simulink model "orthosis_robust"  (R2017b)
settings: Solver=ode45  StartTime=0.0  StopTime=40  RelTol=1e-3
settings Model: SimulationMode=accelerator  Creator=ArsalanBangash  LastModifiedBy=ArsalanBangash

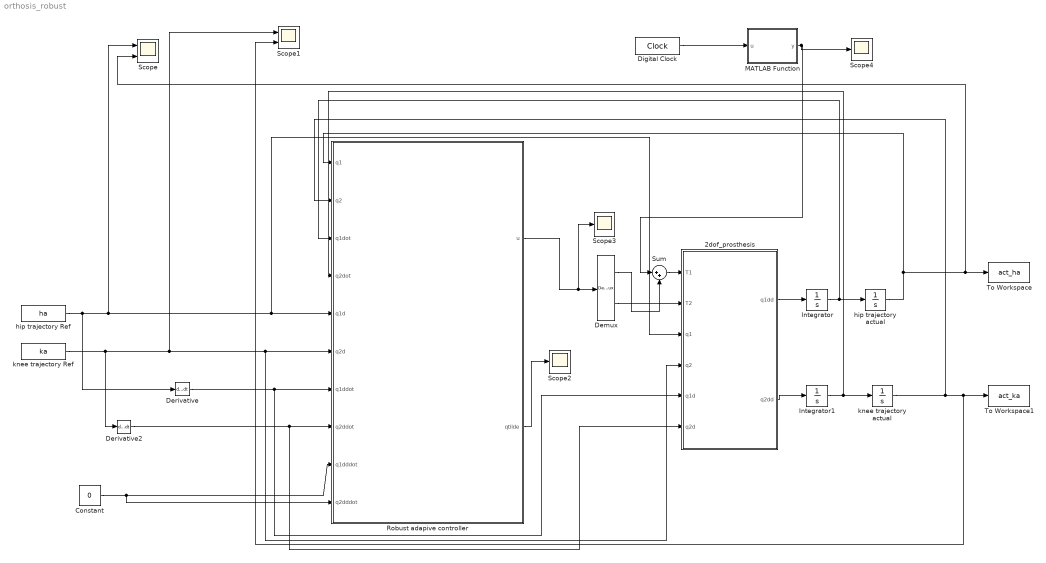
== system orthosis_robust ==
  2dof_prosthesis : MATLAB Function  TreatAsAtomicUnit=on
  Constant : Constant  Value=0
  Demux : Demux  Outputs=2
  Derivative : Derivative
  Derivative2 : Derivative
  Digital Clock : DigitalClock
  Integrator : Integrator
  Integrator1 : Integrator
  MATLAB Function : MATLAB Function  TreatAsAtomicUnit=on
  Robust adapive controller : MATLAB Function  TreatAsAtomicUnit=on
  Scope : Scope  NumInputPorts=2
  Scope1 : Scope  NumInputPorts=2
  Scope2 : Scope
  Scope3 : Scope
  Scope4 : Scope
  Sum : Sum  Inputs=|++
  To Workspace : ToWorkspace  VariableName=act_ha  SampleTime=-1
  To Workspace1 : ToWorkspace  VariableName=act_ka  SampleTime=-1
  hip trajectory Ref : FromWorkspace  VariableName=ha  SampleTime=0
  hip trajectory actual : Integrator
  knee trajectory Ref : FromWorkspace  VariableName=ka  SampleTime=0
  knee trajectory actual : Integrator
  wires:
  2dof_prosthesis/1(q1dd) -> Integrator/1
  knee trajectory actual/1 -> Robust adapive controller/2(q2), Scope1/2, To Workspace1/1
  Demux/2 -> 2dof_prosthesis/2(T2)
  Constant/1 -> Robust adapive controller/10(q2dddot), Robust adapive controller/9(q1dddot)
  Integrator/1 -> Robust adapive controller/3(q1dot), hip trajectory actual/1
  2dof_prosthesis/2(q2dd) -> Integrator1/1
  hip trajectory Ref/1 -> Scope/1, 2dof_prosthesis/3(q1), Robust adapive controller/5(q1d), Derivative/1
  Integrator1/1 -> Robust adapive controller/4(q2dot), knee trajectory actual/1
  knee trajectory Ref/1 -> Scope1/1, 2dof_prosthesis/4(q2), Robust adapive controller/6(q2d), Derivative2/1
  hip trajectory actual/1 -> Robust adapive controller/1(q1), Scope/2, To Workspace/1
  Derivative/1 -> 2dof_prosthesis/5(q1d), Robust adapive controller/7(q1ddot)
  Derivative2/1 -> 2dof_prosthesis/6(q2d), Robust adapive controller/8(q2ddot)
  Robust adapive controller/1(u) -> Scope3/1, Demux/1
  Robust adapive controller/2(qtilde) -> Scope2/1
  Digital Clock/1 -> MATLAB Function/1(u)
  Demux/1 -> Sum/2
  MATLAB Function/1(y) -> Scope4/1, Sum/1
  Sum/1 -> 2dof_prosthesis/1(T1)

== matlab function orthosis_robust/MATLAB Function ==
  data: u input; y output
function y= fcn(u)
time=u;
if (time>10 && time<20)
    y=200;
else
    y=0;
end

== matlab function orthosis_robust/Robust adapive controller ==
  data: q1 input; u output; q2 input; q1dot input; q2dot input; q1d input; q2d input; q1ddot input; q2ddot input; q1dddot input; q2dddot input; qtilde output
function [u,qtilde]=robust_passivity(q1,q2,q1dot,q2dot,q1d,q2d,q1ddot,q2ddot,q1dddot,q2dddot)
%In-class example: 2-link planar RR manipulator
g=9.8;
qtilde=[q1-q1d;q2-q2d];
qtildedot=[q1dot-q1ddot;q2dot-q2ddot];

%Gains
L=diag([1 1]);
K=diag([1 1]);

v=[q1ddot;q2ddot]-L*qtilde;
a=[q1dddot;q2dddot]-L*qtildedot;
r=qtildedot+L*qtilde;

%Form the regressor
Y=zeros(2,5);
Y(1,1)=a(1);
Y(1,2)=cos(q2)*(2*a(1)+a(2))-sin(q2)*q2dot*v(1)-sin(q2)*(q1dot+q2dot)*v(2);
Y(1,3)=a(2);
Y(1,4)=g*cos(q1);
Y(1,5)=g*cos(q1+q2);
Y(2,1)=0;
Y(2,2)=cos(q2)*a(1)+sin(q2)*q1dot*v(1);
Y(2,3)=a(1)+a(2);
Y(2,4)=0;
Y(2,5)=Y(1,5);

TH_0=[42.1;0.96;12.32;7.8;3.2];

deadzone=0.1;
rho=5.6158;
s=Y'*r;
if norm(s)>deadzone,
    dTh=-rho*s/norm(s);
else
    dTh=[0;0;0;0;0];
end
Th_hat=TH_0+dTh;

u=Y*Th_hat-K*r;

== matlab function orthosis_robust/2dof_prosthesis ==
  data: T1 input; q1dd output; T2 input; q2dd output; q1 input; q2 input; q1d input; q2d input
function [q1dd,q2dd]= fcn(T1, T2,q1,q2,q1d,q2d)


m1=1;
m2=1;
l1=1;
l2=1;
g0=9.8;
Ixx1=0.00205024; Ixx2=0.00205024;Iyy1=0.00205024;Iyy2=0.00205024;
Izz1=0.00205024; Izz2=0.00205024;

B=[ Izz1 + Izz2 + 0.25*l1^2*m1 + l1^2*m2 + 0.25*l2^2*m2 + l1*l2*m2*cos(q2), 0.25*m2*l2^2 + 0.5*l1*m2*cos(q2)*l2 + Izz2;
                             0.25*m2*l2^2 + 0.5*l1*m2*cos(q2)*l2 + Izz2,                        0.25*m2*l2^2 + Izz2];


C=[ -0.5*l1*l2*m2*q2d*sin(q2), -(l1*l2*m2*sin(q2)*(q1d + q2d))/2;
  0.5*l1*l2*m2*q1d*sin(q2),                                 0];




 G= [1.0*g0*m2*(0.5*l2*cos(q1 + q2) + 1.0*l1*cos(q1)) + 0.5*g0*l1*m1*cos(q1)
                                               0.5*g0*l2*m2*cos(q1 + q2)];
 


T=[T1;T2];

thd=[q1d;
q2d];

actual_th_dd= inv(B)*(T-C*thd-G);
q1dd= actual_th_dd(1);
q2dd=actual_th_dd(2);
